simulink model "model_sim_fuzzy"  (R2024b)
settings: Solver=FixedStepAuto  StartTime=0.0  StopTime=10  FixedStep=0.01  RelTol=1e-3
undefined symbols (not defined in the file): controller
settings Model: Creator=usuario  LastModifiedBy=usuario
settings DataIOCC: ReturnWorkspaceOutputs=off  TimeSaveName=t
settings RTWCC: GPUComputeCapability=3.5

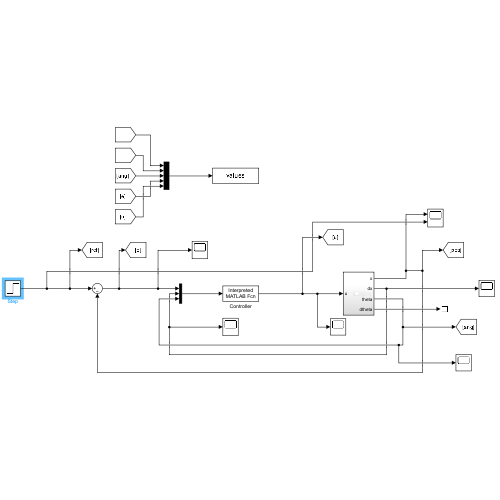
[thumbnail: Simulink's stored preview of the top-level diagram]
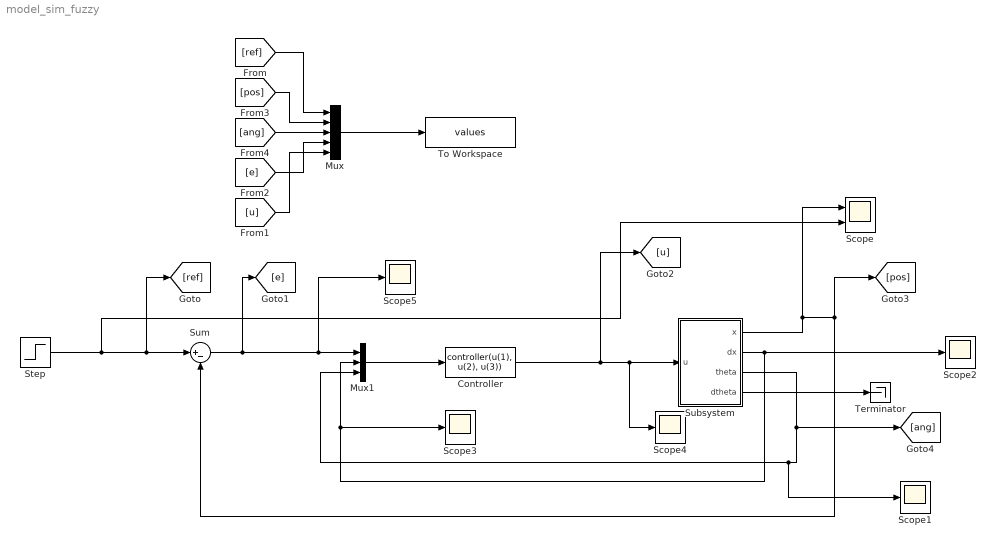
== system model_sim_fuzzy ==
  Controller : MATLABFcn  MATLABFcn=controller(u(1), u(2), u(3))  OutputSignalType=real
  Mux : Mux  Inputs=5
  Mux1 : Mux  Inputs=3
  Scope : Scope  NumInputPorts=2
  Scope{1..5} (5 alike) : Scope
  Step : Step  After=0.6  SampleTime=0
  Subsystem : Subsystem
  Sum : Sum  Inputs=|+-
  Terminator : Terminator
  To Workspace : ToWorkspace  VariableName=values  SampleTime=-1
  wires:
  Mux/1 -> To Workspace/1
  Subsystem/1(x) -> Scope/1, Sum/2, [pos]
  Subsystem/3(theta) -> Scope1/1, Mux1/3, [ang]
  Step/1 -> Scope/2, [ref], Sum/1
  Subsystem/4(dtheta) -> Terminator/1
  [ref] -> Mux/1
  [pos] -> Mux/2
  [ang] -> Mux/3
  [e] -> Mux/4
  [u] -> Mux/5
  Sum/1 -> [e], Scope5/1, Mux1/1
  Subsystem/2(dx) -> Scope3/1, Mux1/2, Scope2/1
  Controller/1 -> [u], Scope4/1, Subsystem/1(u)
  Mux1/1 -> Controller/1

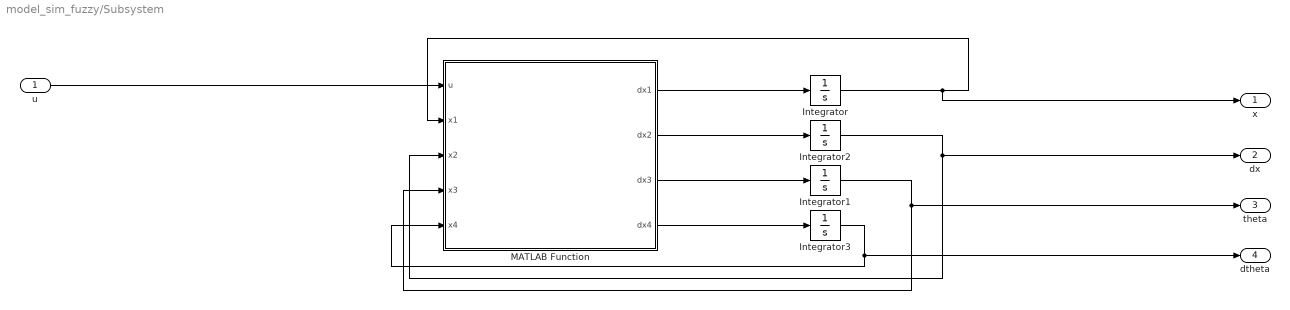
== system model_sim_fuzzy/Subsystem ==
  u : Inport
  Integrator : Integrator  InitialCondition=0.002
  Integrator1 : Integrator  InitialCondition=0.001
  Integrator2 : Integrator
  Integrator3 : Integrator
  MATLAB Function : MATLAB Function  TreatAsAtomicUnit=on
  x : Outport
  dx : Outport  Port=2
  theta : Outport  Port=3
  dtheta : Outport  Port=4
  wires:
  MATLAB Function/2(dx2) -> Integrator2/1
  Integrator/1 -> x/1, MATLAB Function/2(x1)
  Integrator2/1 -> MATLAB Function/3(x2), dx/1
  MATLAB Function/4(dx4) -> Integrator3/1
  MATLAB Function/1(dx1) -> Integrator/1
  MATLAB Function/3(dx3) -> Integrator1/1
  Integrator3/1 -> MATLAB Function/5(x4), dtheta/1
  Integrator1/1 -> theta/1, MATLAB Function/4(x3)
  u/1 -> MATLAB Function/1(u)

== matlab function model_sim_fuzzy/Subsystem/MATLAB Function ==
  data: u input; dx1 output; x1 input; x2 input; x3 input; x4 input; dx2 output; dx3 output; dx4 output
function [dx1,dx2,dx3,dx4] = plant_model(u,x1,x2,x3,x4)
M = 10;g=9.8;m=5;l=1;mu=0.3;
q = [x1;x2;x3;x4];
a11 = -mu/(M+m*sin(x3)^2); a12 = m*g*cos(x3)*sin(x3)/((M+m*sin(x3)^2)*x3);
a13 = m*l*x4*sin(x3)/(M+m*sin(x3)^2); a21 = mu*cos(x3)/(l*(M+m*sin(x3)^2));
a22 = -(M+m)*g*sin(x3)/(l*x3*(M+m*sin(x3)^2)); a23=-m*x4*sin(x3)*cos(x3)/(M+m*sin(x3)^2);
b1 = 1/(M+m*sin(x3)^2); b2 = -cos(x3)/(l*(M+m*sin(x3)^2));
A = [0 1 0 0;0 a11 a12 a13;0 0 0 1;0 a21 a22 a23];
B = [0;b1;0;b2];

dq = A*q + B*u;
dx1 = dq(1);
dx2 = dq(2);
dx3 = dq(3);
dx4 = dq(4);
